simulink model "stp1_confrontation"  (R2022b)
settings: Solver=VariableStepAuto  StartTime=0.0  StopTime=5  RelTol=1e-3
values from neighbouring files (symbols this model uses):
  K = inv(M'*M + lambda*eye(Nu)) * M'    [dmc.m]    (also in dpid.m = 7.7; gpc.m; stp1.m = acker(A, B, [s s s]))
  L = acker(A', C', [s0 s0 s0])    [stp1.m]
  x1_0 = 2    [stp1.m]
  x1_05 = 2    [stp1.m]
  x2_0 = 1    [stp1.m]
  x2_05 = 1    [stp1.m]
  x3_0 = -1    [stp1.m]
  x3_05 = -1    [stp1.m]
  x_ob = [0 0 0]    [stp1.m]
settings Model: Creator=zalew  LastModifiedBy=zalew

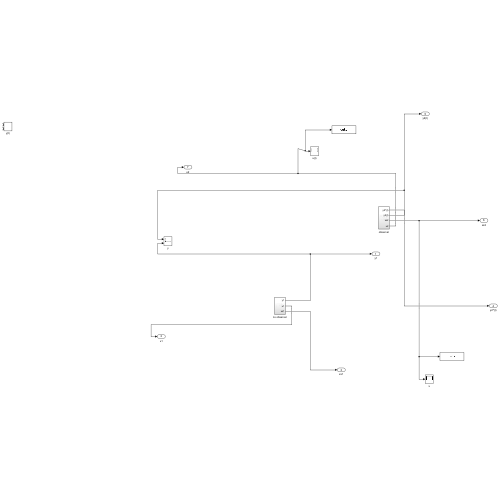
[thumbnail: Simulink's stored preview of the top-level diagram]
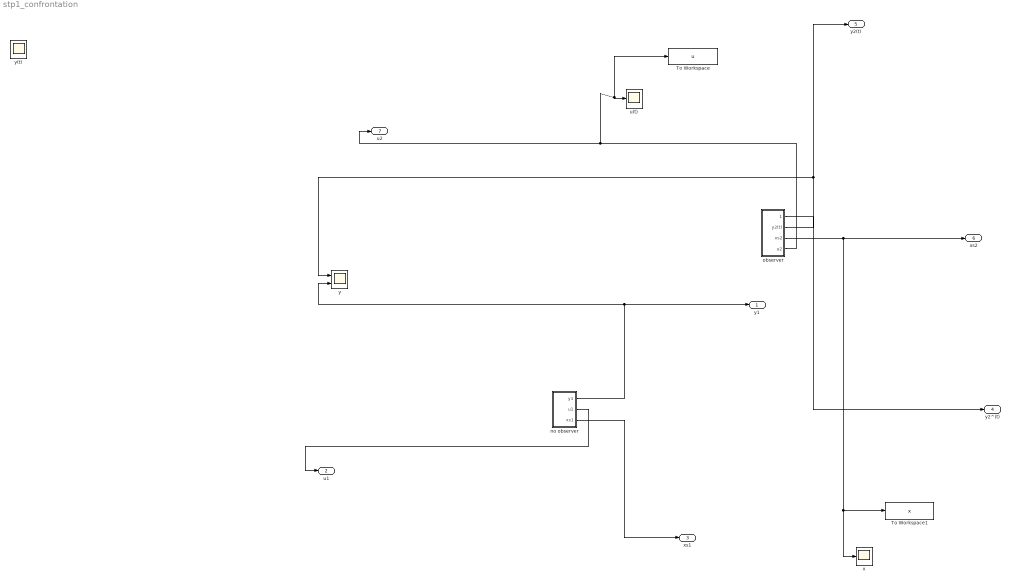
== system stp1_confrontation ==
  To Workspace : ToWorkspace  VariableName=u  SaveFormat=Timeseries  SampleTime=-1
  To Workspace1 : ToWorkspace  VariableName=x  SaveFormat=Timeseries  SampleTime=-1
  no observer : Subsystem
  observer : Subsystem
  u(t) : Scope
  x : Scope
  y : Scope  NumInputPorts=2
  y(t) : Scope  NumInputPorts=2
  y1 : Outport
  u1 : Outport  Port=2
  xs1 : Outport  Port=3
  y2^(t) : Outport  Port=4
  y2(t) : Outport  Port=5
  xs2 : Outport  Port=6
  u2 : Outport  Port=7
  wires:
  no observer/1(y1) -> y1/1, y/2
  no observer/2(u1) -> u1/1
  no observer/3(xs1) -> xs1/1
  observer/4(u2) -> To Workspace/1, u(t)/1, u2/1
  observer/1(y2^(t)) -> y2^(t)/1
  observer/3(xs2) -> xs2/1, x/1, To Workspace1/1
  observer/2(y2(t)) -> y2(t)/1, y/1

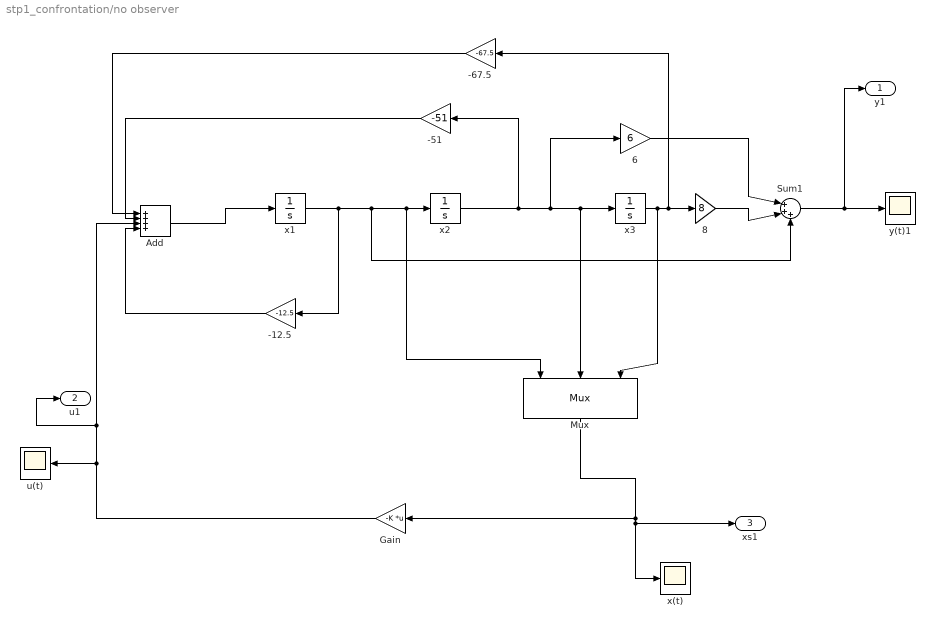
== system stp1_confrontation/no observer ==
  -12.5 : Gain  Gain=-12.5
  -51 : Gain  Gain=-51
  -67.5 : Gain  Gain=-67.5
  6 : Gain  Gain=6
  8 : Gain  Gain=8
  Add : Sum  Inputs=++++
  Gain : Gain  Gain=-K  Multiplication=Matrix(K*u) (u vector)
  Mux : Mux  Inputs=3
      settings: DisplayOption=signals
  Sum1 : Sum  Inputs=|+++
  u(t) : Scope
  x(t) : Scope
  x1 : Integrator  InitialCondition=x1_0
  x2 : Integrator  InitialCondition=x2_0
  x3 : Integrator  InitialCondition=x3_0
  y(t)1 : Scope
  y1 : Outport
  u1 : Outport  Port=2
  xs1 : Outport  Port=3
  wires:
  Gain/1 -> u(t)/1, u1/1, Add/3
  Add/1 -> x1/1
  x1/1 -> -12.5/1, Mux/1, x2/1, Sum1/3
  -67.5/1 -> Add/1
  Mux/1 -> xs1/1, x(t)/1, Gain/1
  Sum1/1 -> y1/1, y(t)1/1
  x3/1 -> Mux/3, -67.5/1, 8/1
  -12.5/1 -> Add/4
  x2/1 -> x3/1, Mux/2, 6/1, -51/1
  -51/1 -> Add/2
  6/1 -> Sum1/1
  8/1 -> Sum1/2

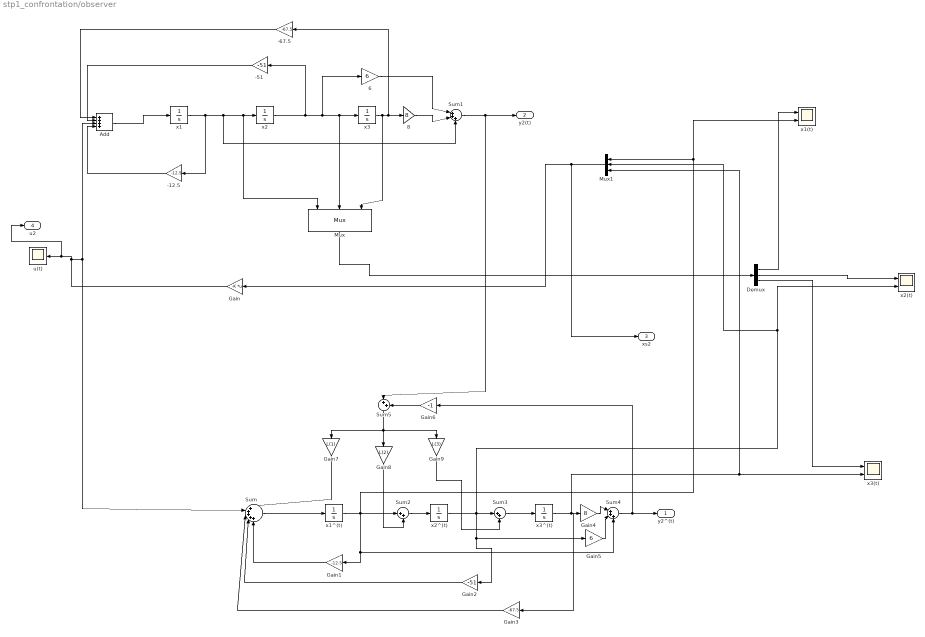
== system stp1_confrontation/observer ==
  -12.5 : Gain  Gain=-12.5
  -51 : Gain  Gain=-51
  -67.5 : Gain  Gain=-67.5
  6 : Gain  Gain=6
  8 : Gain  Gain=8
  Add : Sum  Inputs=++++
  Demux : Demux  Outputs=3
  Gain : Gain  Gain=-K  Multiplication=Matrix(K*u) (u vector)
  Gain1 : Gain  Gain=-12.5
  Gain2 : Gain  Gain=-51
  Gain3 : Gain  Gain=-67.5
  Gain4 : Gain  Gain=8
  Gain5 : Gain  Gain=6
  Gain6 : Gain  Gain=-1
  Gain7 : Gain  Gain=L(1)
  Gain8 : Gain  Gain=L(2)
  Gain9 : Gain  Gain=L(3)
  Mux : Mux  Inputs=3
      settings: DisplayOption=signals
  Mux1 : Mux  Inputs=3
  Sum : Sum  Inputs=|+++++
  Sum1 : Sum  Inputs=|+++
  Sum2 : Sum  Inputs=|++
  Sum3 : Sum  Inputs=|++
  Sum4 : Sum  Inputs=|+++
  Sum5 : Sum  Inputs=|++
  u(t) : Scope
  x1 : Integrator  InitialCondition=x1_05
  x1(t) : Scope  NumInputPorts=2
  x1^(t) : Integrator  InitialCondition=x_ob(1)
  x2 : Integrator  InitialCondition=x2_05
  x2(t) : Scope  NumInputPorts=2
  x2^(t) : Integrator  InitialCondition=x_ob(2)
  x3 : Integrator  InitialCondition=x3_05
  x3(t) : Scope  NumInputPorts=2
  x3^(t) : Integrator  InitialCondition=x_ob(3)
  y2^(t) : Outport
  y2(t) : Outport  Port=2
  xs2 : Outport  Port=3
  u2 : Outport  Port=4
  wires:
  Gain3/1 -> Sum/3
  Mux1/1 -> xs2/1, Gain/1
  Sum4/1 -> y2^(t)/1, Gain6/1
  -12.5/1 -> Add/4
  x2/1 -> x3/1, Mux/2, 6/1, -51/1
  Sum5/1 -> Gain9/1, Gain8/1, Gain7/1
  x3/1 -> Mux/3, -67.5/1, 8/1
  Gain2/1 -> Sum/4
  Add/1 -> x1/1
  x1^(t)/1 -> x1(t)/2, Mux1/1, Sum4/3, Gain1/1, Sum2/1
  Demux/3 -> x3(t)/1
  x1/1 -> -12.5/1, Mux/1, x2/1, Sum1/3
  8/1 -> Sum1/2
  Sum1/1 -> y2(t)/1, Sum5/1
  Gain/1 -> Add/3, Sum/2, u2/1, u(t)/1
  Sum/1 -> x1^(t)/1
  Gain7/1 -> Sum/1
  x2^(t)/1 -> Mux1/2, x2(t)/2, Gain5/1, Gain2/1, Sum3/1
  Mux/1 -> Demux/1
  6/1 -> Sum1/1
  Gain4/1 -> Sum4/1
  -67.5/1 -> Add/1
  Gain1/1 -> Sum/5
  Demux/2 -> x2(t)/1
  Gain9/1 -> Sum3/2
  -51/1 -> Add/2
  Gain8/1 -> Sum2/2
  Sum3/1 -> x3^(t)/1
  Demux/1 -> x1(t)/1
  Gain6/1 -> Sum5/2
  Sum2/1 -> x2^(t)/1
  Gain5/1 -> Sum4/2
  x3^(t)/1 -> x3(t)/2, Mux1/3, Gain3/1, Gain4/1
